simulink model "ABS_EBD"  (R2022b)
settings: Solver=VariableStepAuto  StartTime=0.0  StopTime=60  RelTol=1e-3
values from neighbouring files (symbols this model uses):
  d = 1.5    [ABS_config.m]
  gp = 9.81    [ABS_config.m]
  h = 0.7    [ABS_config.m]
  J = 0.5    [ABS_config.m]
  m = 1000    [ABS_config.m]
  rR = 0.3    [ABS_config.m]
  V0 = 27.77    [ABS_config.m]
  w0 = V0/rR    (= 92.5666666667)    [ABS_config.m]
libraries: simulink x2, slpidlib x2
settings Model: Creator=elmeh  LastModifiedBy=Youssef ABLALI
settings SolverCC: ZeroCrossAlgorithm=Adaptive
settings DebuggingCC: IgnoredZcDiagnostic=none

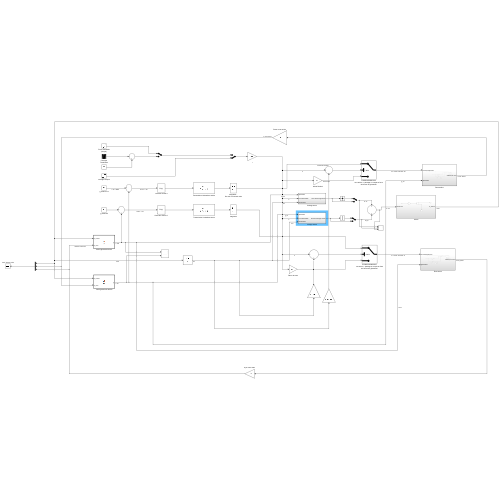
[thumbnail: Simulink's stored preview of the top-level diagram]
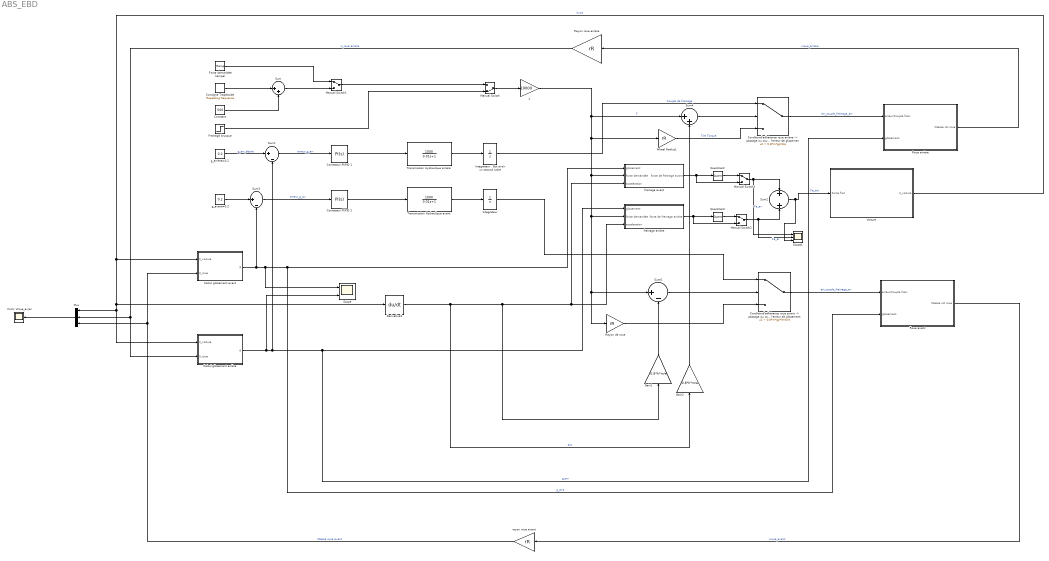
== system ABS_EBD ==
  Calcul glissement arrière : MATLAB Function  TreatAsAtomicUnit=on
  Calcul glissement avant : MATLAB Function  TreatAsAtomicUnit=on
  "Conditiond'adhérence roue arrière -> passage ou couple en fonct de l'erreur de glissemen" : Switch  Criteria=u2 > Threshold  Threshold=0.8*m*gp*d/e  SaturateOnIntegerOverflow=off  InputSameDT=off
  "Conditiond'adhérence roue avant -> passage ou couple en fonct de l'erreur de glissement" : Switch  Criteria=u2 > Threshold  Threshold=0.8*m*gp*(e-d)/e  SaturateOnIntegerOverflow=off  InputSameDT=off
  Consigne Trapézoide : simulink/Sources/Repeating Sequence  rep_seq_t=[0 0.1 0.2 0.3 0.4 0.5]  rep_seq_y=[0 1000 1000 1000 0 0]
  Constant : Constant  Value=500
  Correcteur PI/PID 1 : slpidlib/PID Controller  Controller=PI  Form=Parallel  TimeDomain=Continuous-time  UseExternalTs=off  SampleTime=-1  IntegratorMethod=Forward Euler  FilterMethod=Forward Euler  ControllerParametersSource=internal  P=50  I=0.2  UseKiTs=off  D=0.001  N=100  UseFilter=on  TunerSelectOption=Transfer Function Based (PID Tuner App)  InitialConditionSource=internal  InitialConditionForIntegrator=0  InitialConditionForFilter=0  DifferentiatorICPrevScaledInput=0  ExternalReset=none  TrackingMode=off  Kt=1  LimitOutput=off  SatLimitsSource=internal  UpperSaturationLimit=inf  LowerSaturationLimit=-inf  LinearizeAsGain=on  AntiWindupMode=none  Kb=1  LimitIntegrator=off  UpperIntegratorSaturationLimit=inf  LowerIntegratorSaturationLimit=-inf  POutMin=[]  POutMax=[]  IOutMin=[]  IOutMax=[]  DOutMin=[]  DOutMax=[]  NOutMin=[]  NOutMax=[]  SumOutMin=[]  SumOutMax=[]  SaturationOutMin=[]  SaturationOutMax=[]  PParamMin=[]  PParamMax=[]  IParamMin=[]  IParamMax=[]  DParamMin=[]  DParamMax=[]  NParamMin=[]  NParamMax=[]  KbParamMin=[]  KbParamMax=[]  KtParamMin=[]  KtParamMax=[]  KbOutMin=[]  KbOutMax=[]  KtOutMin=[]  KtOutMax=[]  IntegratorOutMin=[]  IntegratorOutMax=[]  FilterOutMin=[]  FilterOutMax=[]  SumI1OutMin=[]  SumI1OutMax=[]  SumI2OutMin=[]  SumI2OutMax=[]  SumI3OutMin=[]  SumI3OutMax=[]  SumI4OutMin=[]  SumI4OutMax=[]  SumDOutMin=[]  SumDOutMax=[]  DifferentiatorOutMin=[]  DifferentiatorOutMax=[]  FilterDiffOutCoefMin=[]  FilterDiffOutCoefMax=[]  ReciprocalOutMin=[]  ReciprocalOutMax=[]  SumDenOutMin=[]  SumDenOutMax=[]  SumNumOutMin=[]  SumNumOutMax=[]  DivideOutMin=[]  DivideOutMax=[]  UdiffTsProdOutMin=[]  UdiffTsProdOutMax=[]  NTsProdOutMin=[]  NTsProdOutMax=[]  UintegralTsProdOutMin=[]  UintegralTsProdOutMax=[]  UngainTsProdOutMin=[]  UngainTsProdOutMax=[]  ClampingZeroOutDataTypeStr=Inherit: Inherit via back propagation  ClampingZeroOutMin=[]  ClampingZeroOutMax=[]  FilterDenConstantOutDataTypeStr=Inherit: Inherit via back propagation  FilterDenConstantOutMin=[]  FilterDenConstantOutMax=[]  PCopyOutDataTypeStr=Inherit: Inherit via back propagation  PCopyOutMin=[]  PCopyOutMax=[]  NCopyOutDataTypeStr=Inherit: Inherit via back propagation  NCopyOutMin=[]  NCopyOutMax=[]  IntegratorContinuousStateAttributes=''  IntegratorStateMustResolveToSignalObject=off  IntegratorRTWStateStorageClass=Auto  FilterContinuousStateAttributes=''  FilterStateMustResolveToSignalObject=off  FilterRTWStateStorageClass=Auto  ParallelPVariant=InternalParameters  IdealPVariant=Disabled  IVariant=InternalParameters  DVariant=Disabled  IntegratorVariant=Continuous  SatVariant=Disabled  AWVariant=Passthrough  PCopyVariant=Disabled  TRVariant=Disabled  FdbkBlocksVariant=Forward  IdealPFdbkVariant=Disabled  SatFdbkVariant=Disabled  DerivativeFilterVariant=Disabled  NVariant=Disabled  NCopyVariant=Disabled_SignalSpec  FilterICVariant=Disabled  IntegratorICVariant=InternalICs  ExternalResetVariant=Disabled  TRSumVariant=Passthrough  SumFdbkVariant=Disabled  SumVariant=Sum_PI  TsampFilterVariant=InternalTs  TsampNgainVariant=Passthrough  TsampIntegralVariant=Passthrough  ExternalSaturationOutDataTypeStr=Inherit: Same as second input
  "Correcteur PI/PID 2 " : slpidlib/PID Controller  Controller=PI  Form=Parallel  TimeDomain=Continuous-time  UseExternalTs=off  SampleTime=-1  IntegratorMethod=Forward Euler  FilterMethod=Forward Euler  ControllerParametersSource=internal  P=100  I=1  UseKiTs=off  D=0.001  N=100  UseFilter=on  TunerSelectOption=Transfer Function Based (PID Tuner App)  InitialConditionSource=internal  InitialConditionForIntegrator=0  InitialConditionForFilter=0  DifferentiatorICPrevScaledInput=0  ExternalReset=none  TrackingMode=off  Kt=1  LimitOutput=off  SatLimitsSource=internal  UpperSaturationLimit=inf  LowerSaturationLimit=-inf  LinearizeAsGain=on  AntiWindupMode=none  Kb=1  LimitIntegrator=off  UpperIntegratorSaturationLimit=inf  LowerIntegratorSaturationLimit=-inf  POutMin=[]  POutMax=[]  IOutMin=[]  IOutMax=[]  DOutMin=[]  DOutMax=[]  NOutMin=[]  NOutMax=[]  SumOutMin=[]  SumOutMax=[]  SaturationOutMin=[]  SaturationOutMax=[]  PParamMin=[]  PParamMax=[]  IParamMin=[]  IParamMax=[]  DParamMin=[]  DParamMax=[]  NParamMin=[]  NParamMax=[]  KbParamMin=[]  KbParamMax=[]  KtParamMin=[]  KtParamMax=[]  KbOutMin=[]  KbOutMax=[]  KtOutMin=[]  KtOutMax=[]  IntegratorOutMin=[]  IntegratorOutMax=[]  FilterOutMin=[]  FilterOutMax=[]  SumI1OutMin=[]  SumI1OutMax=[]  SumI2OutMin=[]  SumI2OutMax=[]  SumI3OutMin=[]  SumI3OutMax=[]  SumI4OutMin=[]  SumI4OutMax=[]  SumDOutMin=[]  SumDOutMax=[]  DifferentiatorOutMin=[]  DifferentiatorOutMax=[]  FilterDiffOutCoefMin=[]  FilterDiffOutCoefMax=[]  ReciprocalOutMin=[]  ReciprocalOutMax=[]  SumDenOutMin=[]  SumDenOutMax=[]  SumNumOutMin=[]  SumNumOutMax=[]  DivideOutMin=[]  DivideOutMax=[]  UdiffTsProdOutMin=[]  UdiffTsProdOutMax=[]  NTsProdOutMin=[]  NTsProdOutMax=[]  UintegralTsProdOutMin=[]  UintegralTsProdOutMax=[]  UngainTsProdOutMin=[]  UngainTsProdOutMax=[]  ClampingZeroOutDataTypeStr=Inherit: Inherit via back propagation  ClampingZeroOutMin=[]  ClampingZeroOutMax=[]  FilterDenConstantOutDataTypeStr=Inherit: Inherit via back propagation  FilterDenConstantOutMin=[]  FilterDenConstantOutMax=[]  PCopyOutDataTypeStr=Inherit: Inherit via back propagation  PCopyOutMin=[]  PCopyOutMax=[]  NCopyOutDataTypeStr=Inherit: Inherit via back propagation  NCopyOutMin=[]  NCopyOutMax=[]  IntegratorContinuousStateAttributes=''  IntegratorStateMustResolveToSignalObject=off  IntegratorRTWStateStorageClass=Auto  FilterContinuousStateAttributes=''  FilterStateMustResolveToSignalObject=off  FilterRTWStateStorageClass=Auto  ParallelPVariant=InternalParameters  IdealPVariant=Disabled  IVariant=InternalParameters  DVariant=Disabled  IntegratorVariant=Continuous  SatVariant=Disabled  AWVariant=Passthrough  PCopyVariant=Disabled  TRVariant=Disabled  FdbkBlocksVariant=Forward  IdealPFdbkVariant=Disabled  SatFdbkVariant=Disabled  DerivativeFilterVariant=Disabled  NVariant=Disabled  NCopyVariant=Disabled_SignalSpec  FilterICVariant=Disabled  IntegratorICVariant=InternalICs  ExternalResetVariant=Disabled  TRSumVariant=Passthrough  SumFdbkVariant=Disabled  SumVariant=Sum_PI  TsampFilterVariant=InternalTs  TsampNgainVariant=Passthrough  TsampIntegralVariant=Passthrough  ExternalSaturationOutDataTypeStr=Inherit: Same as second input
  Derivative3 : Derivative
  Force demandée (rampe) : simulink/Sources/Ramp  slope=1  start=0  InitialOutput=0
  Freinage brusque : Step  SampleTime=0
  Gain1 : Gain  Gain=0.8*h*m/e
  Gain2 : Gain  Gain=0.8*h*m/e
  "Integrateur " : Integrator  LimitOutput=on  UpperSaturationLimit=1500  LowerSaturationLimit=0
  "Integrateur : But avoir un second ordre" : Integrator  LimitOutput=on  UpperSaturationLimit=1500  LowerSaturationLimit=0
  Manual Switch : ManualSwitch  CurrentSetting=0
  Manual Switch1 : ManualSwitch
  Manual Switch2 : ManualSwitch
  Manual Switch3 : ManualSwitch
  Mux : Mux  Inputs=3
  Quantizer2 : Quantizer  QuantizationInterval=400
  Quantizer3 : Quantizer  QuantizationInterval=400
  Rayon de roue : Gain  Gain=rR
  Rayon roue arrière : Gain  Gain=rR
  Roue arrière : Subsystem
  Roue avant : Subsystem
  Scope : Scope  NumInputPorts=2
  Scope1 : Scope  NumInputPorts=3
  Sum : Sum  Inputs=|++
  Sum1 : Sum  Inputs=|+-
  Sum2 : Sum  Inputs=+|+
  Sum3 : Sum  Inputs=|+-
  Sum4 : Sum  Inputs=|++
  Sum6 : Sum  Inputs=|+-
  Transmission Hydraulique arrière : TransferFcn  Numerator=[1000]  Denominator=[0.01 1]
  Transmission Hydraulique avant : TransferFcn  Numerator=[1000]  Denominator=[0.01 1]
  Voiture : Subsystem
  "Vvoit, Vroue_av/ar" : Scope
  Wheel Radius1 : Gain  Gain=rR
  "freinage arrière " : Subsystem
  "freinage avant " : Subsystem
  g_arrière=0.2 : Constant  Value=0.2
  g_avant=0.2 : Constant  Value=0.2
  k : Gain  Gain=10000
  rayon roue avant : Gain  Gain=rR
  wires:
  Force demandée (rampe)/1 -> Manual Switch1/1
  Freinage brusque/1 -> Manual Switch/2
  Manual Switch1/1 -> Manual Switch/1
  Sum/1 -> Manual Switch1/2
  Manual Switch/1 -> k/1
  rayon roue avant/1 -> Mux/3, Calcul glissement avant/2(V_roue)  "Vitesse roue avant"
  k/1 -> Sum4/1, Wheel Radius1/1, "freinage arrière "/2(force demandée), Sum6/1, Rayon de roue/1, "freinage avant "/2(force demandée)  "F"
  Consigne Trapézoide/1 -> Sum/1
  Constant/1 -> Sum/2
  g_arrière=0.2/1 -> Sum1/1  "g_arr_désiré"
  Sum1/1 -> Correcteur PI/PID 1/1  "erreur_g_arr"
  "Conditiond'adhérence roue arrière -> passage ou couple en fonct de l'erreur de glissemen"/1 -> Roue arrière/1(erreur/Couple frein)  "err_couple_freinage_arr"
  Transmission Hydraulique arrière/1 -> "Integrateur : But avoir un second ordre"/1
  "Integrateur : But avoir un second ordre"/1 -> "Conditiond'adhérence roue arrière -> passage ou couple en fonct de l'erreur de glissemen"/1  "Couple de freinage"
  Correcteur PI/PID 1/1 -> Transmission Hydraulique arrière/1
  Gain2/1 -> Sum4/2
  Sum4/1 -> "Conditiond'adhérence roue arrière -> passage ou couple en fonct de l'erreur de glissemen"/2
  Wheel Radius1/1 -> "Conditiond'adhérence roue arrière -> passage ou couple en fonct de l'erreur de glissemen"/3  "Tire Torque"
  Manual Switch3/1 -> Scope1/1, Sum2/1  "Fa_av"
  "freinage arrière "/1(force de freinage arrière) -> Manual Switch2/2, Quantizer3/1
  Manual Switch2/1 -> Scope1/2, Sum2/2  "Fa_ar"
  Quantizer3/1 -> Manual Switch2/1
  Quantizer2/1 -> Manual Switch3/1
  "freinage avant "/1(force de freinage avant) -> Manual Switch3/2, Quantizer2/1
  Sum2/1 -> Scope1/3, Voiture/1(Force frot)  "Fa_tot"
  "Integrateur "/1 -> "Conditiond'adhérence roue avant -> passage ou couple en fonct de l'erreur de glissement"/1
  g_avant=0.2/1 -> Sum3/1
  "Correcteur PI/PID 2 "/1 -> Transmission Hydraulique avant/1
  Sum3/1 -> "Correcteur PI/PID 2 "/1  "erreur_g_av"
  Transmission Hydraulique avant/1 -> "Integrateur "/1
  Rayon de roue/1 -> "Conditiond'adhérence roue avant -> passage ou couple en fonct de l'erreur de glissement"/3
  Sum6/1 -> "Conditiond'adhérence roue avant -> passage ou couple en fonct de l'erreur de glissement"/2
  Gain1/1 -> Sum6/2
  "Conditiond'adhérence roue avant -> passage ou couple en fonct de l'erreur de glissement"/1 -> Roue avant/1(erreur/Couple frein)  "err_couple_freinage_av"
  Roue arrière/1(Vitesse rot roue) -> Rayon roue arrière/1  "vroue_arrière"
  Rayon roue arrière/1 -> Mux/2, Calcul glissement arrière/2(V_roue)  "V_roue arrière"
  Voiture/1("V_voiture ") -> Calcul glissement avant/1(V_voiture), Derivative3/1, Mux/1, Calcul glissement arrière/1(V_voiture)  "Vvoit"
  Calcul glissement arrière/1(g) -> Scope/2, Sum1/2, Roue arrière/2(glissement), "freinage arrière "/1("glissement ")  "g_arr"
  Calcul glissement avant/1(g) -> Scope/1, Roue avant/2(glissement), "freinage avant "/1("glissement "), Sum3/2  "g_ava"
  Derivative3/1 -> Gain2/1, Gain1/1, "freinage avant "/3(acceleration), "freinage arrière "/3(acceleration)  "acc"
  Roue avant/1(Vitesse rot roue) -> rayon roue avant/1  "vroue_avant"
  Mux/1 -> "Vvoit, Vroue_av/ar"/1

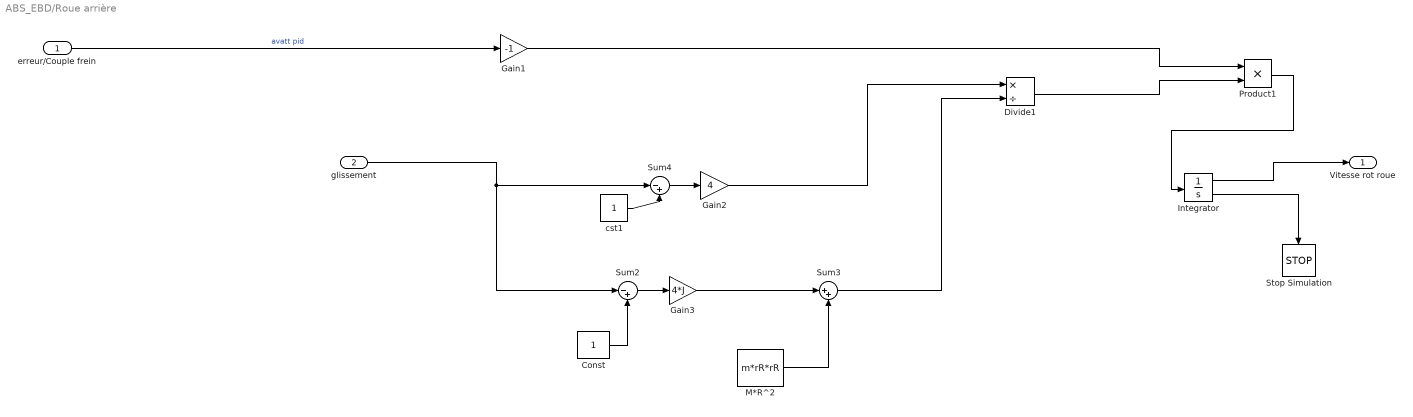
== system ABS_EBD/Roue arrière ==
  erreur/Couple frein : Inport
  glissement : Inport  Port=2
  Const : Constant
  Divide1 : Product  Inputs=*/
  Gain1 : Gain  Gain=-1
  Gain2 : Gain  Gain=4
  Gain3 : Gain  Gain=4*J
  Integrator : Integrator  InitialCondition=w0  LimitOutput=on  LowerSaturationLimit=0  ShowSaturationPort=on
  M*R^2 : Constant  Value=m*rR*rR
  Product1 : Product
  Stop Simulation : Stop
  Sum2 : Sum  Inputs=|-+
  Sum3 : Sum  Inputs=|++
  Sum4 : Sum  Inputs=|-+
  cst1 : Constant
  Vitesse rot roue : Outport
  wires:
  Integrator/2 -> Stop Simulation/1
  Product1/1 -> Integrator/1
  glissement/1 -> Sum2/1, Sum4/1
  Const/1 -> Sum2/2
  M*R^2/1 -> Sum3/2
  Sum3/1 -> Divide1/2
  Gain2/1 -> Divide1/1
  Gain1/1 -> Product1/1
  Sum2/1 -> Gain3/1
  Sum4/1 -> Gain2/1
  Divide1/1 -> Product1/2
  Gain3/1 -> Sum3/1
  cst1/1 -> Sum4/2
  Integrator/1 -> Vitesse rot roue/1
  erreur/Couple frein/1 -> Gain1/1  "avatt pid"

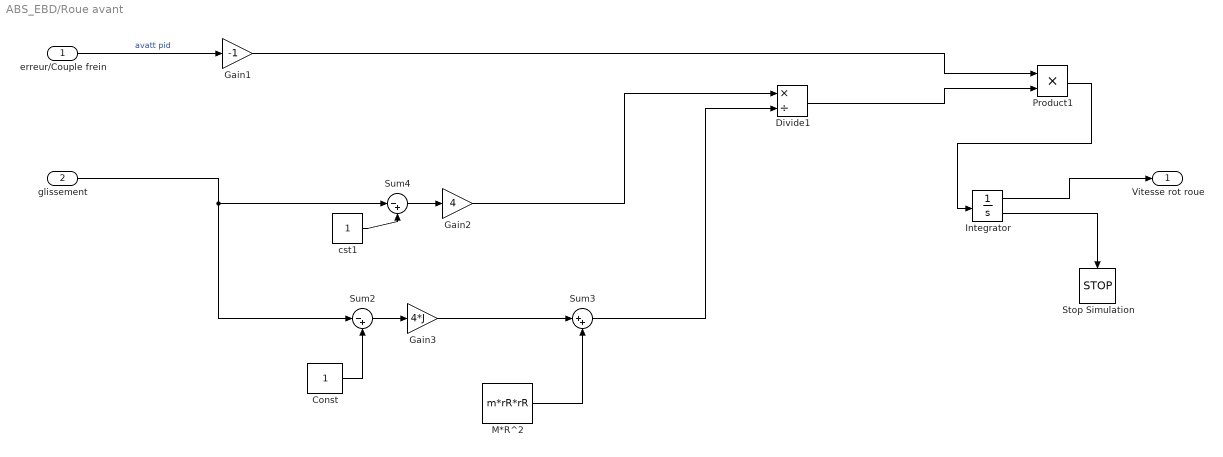
== system ABS_EBD/Roue avant ==
  erreur/Couple frein : Inport
  glissement : Inport  Port=2
  Const : Constant
  Divide1 : Product  Inputs=*/
  Gain1 : Gain  Gain=-1
  Gain2 : Gain  Gain=4
  Gain3 : Gain  Gain=4*J
  Integrator : Integrator  InitialCondition=w0  LimitOutput=on  LowerSaturationLimit=0  ShowSaturationPort=on
  M*R^2 : Constant  Value=m*rR*rR
  Product1 : Product
  Stop Simulation : Stop
  Sum2 : Sum  Inputs=|-+
  Sum3 : Sum  Inputs=|++
  Sum4 : Sum  Inputs=|-+
  cst1 : Constant
  Vitesse rot roue : Outport
  wires:
  Integrator/2 -> Stop Simulation/1
  Product1/1 -> Integrator/1
  glissement/1 -> Sum2/1, Sum4/1
  Const/1 -> Sum2/2
  M*R^2/1 -> Sum3/2
  Sum3/1 -> Divide1/2
  Gain2/1 -> Divide1/1
  Gain1/1 -> Product1/1
  Sum2/1 -> Gain3/1
  Sum4/1 -> Gain2/1
  Divide1/1 -> Product1/2
  Gain3/1 -> Sum3/1
  cst1/1 -> Sum4/2
  Integrator/1 -> Vitesse rot roue/1
  erreur/Couple frein/1 -> Gain1/1  "avatt pid"

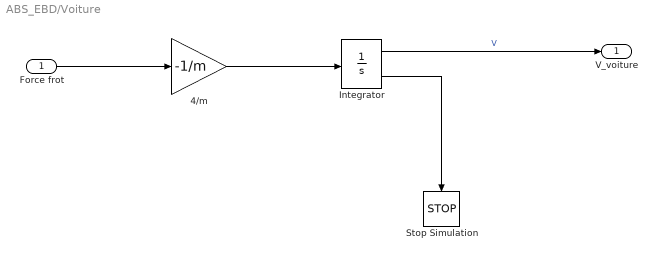
== system ABS_EBD/Voiture ==
  Force frot : Inport
  4/m : Gain  Gain=-1/m
  Integrator : Integrator  InitialCondition=V0  LimitOutput=on  LowerSaturationLimit=0  ShowSaturationPort=on
  Stop Simulation : Stop
  "V_voiture " : Outport
  wires:
  Force frot/1 -> 4/m/1
  4/m/1 -> Integrator/1
  Integrator/1 -> "V_voiture "/1  "V"
  Integrator/2 -> Stop Simulation/1

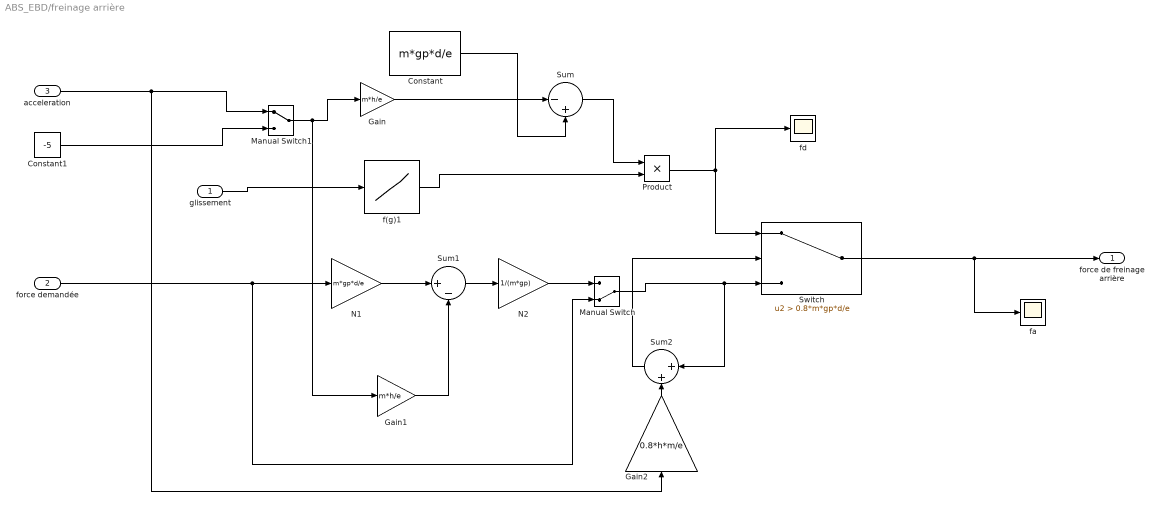
== system ABS_EBD/freinage arrière  ==
  "glissement " : Inport
  force demandée : Inport  Port=2
  acceleration : Inport  Port=3
  Constant : Constant  Value=m*gp*d/e
  Constant1 : Constant  Value=-5
  Gain : Gain  Gain=m*h/e
  Gain1 : Gain  Gain=m*h/e
  Gain2 : Gain  Gain=0.8*h*m/e
  Manual Switch : ManualSwitch  CurrentSetting=0
  Manual Switch1 : ManualSwitch
  N1 : Gain  Gain=m*gp*d/e
  N2 : Gain  Gain=1/(m*gp)
  Product : Product
  Sum : Sum  Inputs=|-+
  Sum1 : Sum  Inputs=|+-
  Sum2 : Sum  Inputs=|++
  Switch : Switch  Criteria=u2 > Threshold  Threshold=0.8*m*gp*d/e  SaturateOnIntegerOverflow=off  InputSameDT=off
  f(g)1 : Lookup_n-D  NumberOfTableDimensions=1  BreakpointsForDimension1=[0,0.1,0.2,0.3,0.4,0.5,0.6,0.7,0.8,0.9,1.0]  Table=[0,0.85,0.95,0.78,0.73,0.7,0.68,0.66,0.64,0.62,0.61]  InternalRulePriority=Speed  RndMeth=Simplest
  fa : Scope
  fd : Scope
  force de freinage arrière : Outport  VectorParamsAs1DForOutWhenUnconnected=off
  wires:
  Switch/1 -> force de freinage arrière/1, fa/1
  "glissement "/1 -> f(g)1/1
  force demandée/1 -> Manual Switch/2, N1/1
  Gain/1 -> Sum/1
  Constant/1 -> Sum/2
  N1/1 -> Sum1/1
  Manual Switch/1 -> Sum2/1, Switch/3
  Gain1/1 -> Sum1/2
  Sum1/1 -> N2/1
  N2/1 -> Manual Switch/1
  Sum/1 -> Product/1
  f(g)1/1 -> Product/2
  Product/1 -> Switch/1, fd/1
  Constant1/1 -> Manual Switch1/2
  Manual Switch1/1 -> Gain1/1, Gain/1
  Gain2/1 -> Sum2/2
  Sum2/1 -> Switch/2
  acceleration/1 -> Gain2/1, Manual Switch1/1

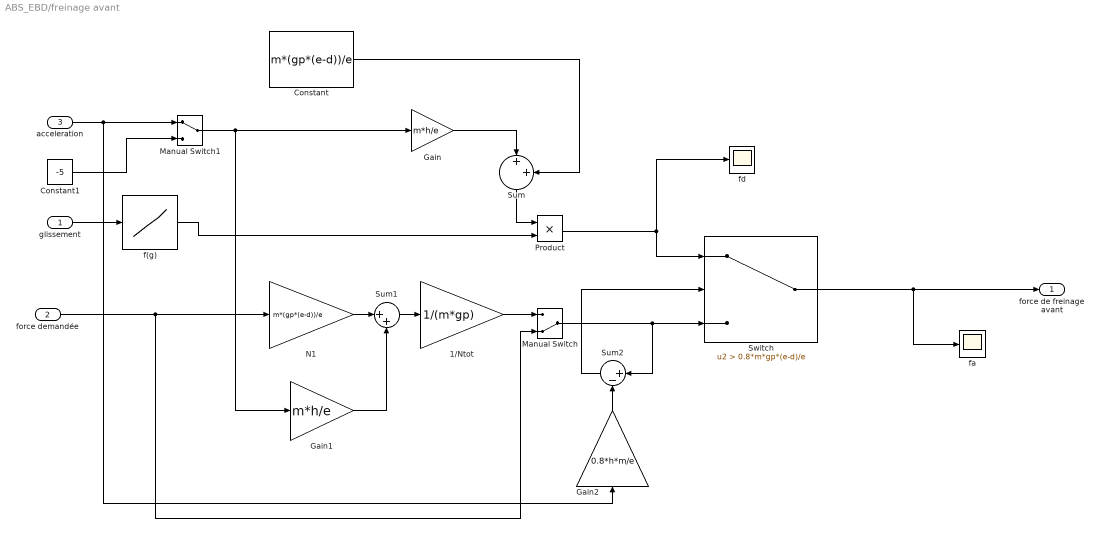
== system ABS_EBD/freinage avant  ==
  "glissement " : Inport
  force demandée : Inport  Port=2
  acceleration : Inport  Port=3
  1/Ntot : Gain  Gain=1/(m*gp)
  Constant : Constant  Value=m*(gp*(e-d))/e
  Constant1 : Constant  Value=-5
  Gain : Gain  Gain=m*h/e
  Gain1 : Gain  Gain=m*h/e
  Gain2 : Gain  Gain=0.8*h*m/e
  Manual Switch : ManualSwitch  CurrentSetting=0
  Manual Switch1 : ManualSwitch
  N1 : Gain  Gain=m*(gp*(e-d))/e
  Product : Product
  Sum : Sum  Inputs=|++
  Sum1 : Sum  Inputs=|++
  Sum2 : Sum  Inputs=|+-
  Switch : Switch  Criteria=u2 > Threshold  Threshold=0.8*m*gp*(e-d)/e  SaturateOnIntegerOverflow=off  InputSameDT=off
  f(g) : Lookup_n-D  NumberOfTableDimensions=1  BreakpointsForDimension1=[0,0.1,0.2,0.3,0.4,0.5,0.6,0.7,0.8,0.9,1.0]  Table=[0,0.85,0.95,0.78,0.73,0.7,0.68,0.66,0.64,0.62,0.61]  InternalRulePriority=Speed  RndMeth=Simplest
  fa : Scope
  fd : Scope
  force de freinage avant : Outport  VectorParamsAs1DForOutWhenUnconnected=off
  wires:
  Switch/1 -> fa/1, force de freinage avant/1
  "glissement "/1 -> f(g)/1
  f(g)/1 -> Product/2
  Constant/1 -> Sum/2
  force demandée/1 -> Manual Switch/2, N1/1
  Gain/1 -> Sum/1
  N1/1 -> Sum1/1
  Manual Switch/1 -> Switch/3, Sum2/1
  Gain1/1 -> Sum1/2
  Sum1/1 -> 1/Ntot/1
  1/Ntot/1 -> Manual Switch/1
  Sum/1 -> Product/1
  Product/1 -> fd/1, Switch/1
  Manual Switch1/1 -> Gain1/1, Gain/1
  Constant1/1 -> Manual Switch1/2
  acceleration/1 -> Gain2/1, Manual Switch1/1
  Gain2/1 -> Sum2/2
  Sum2/1 -> Switch/2

== matlab function ABS_EBD/Calcul glissement avant ==
  data: V_voiture input; V_roue input; g output
function g = fcn(V_voiture,V_roue)

g = (V_voiture - V_roue)/V_voiture;

== matlab function ABS_EBD/Calcul glissement arrière ==
  data: V_voiture input; V_roue input; g output
function g = fcn(V_voiture,V_roue)

g = (V_voiture - V_roue)/V_voiture;
